simulink model "test_interp_method"  (R2025a)
settings: Solver=FixedStepAuto  StartTime=0.0  StopTime=.01  FixedStep=0.005  RelTol=1e-3
values from neighbouring files (symbols this model uses):
  SimIn =     [Model+Units_TEST.mat]    (also in SimIn_FROZEN.mat)
  ubar_cmd = 0.5 * (XU0_interp(1,4,2) + XU0_interp(1,3,2))    [config_and_run_interp_method_test.m]
  wbar_cmd = XU0_interp(3,3,2)    [config_and_run_interp_method_test.m]
libraries: simulink_extras x23
settings Model: Creator=alhallmark  LastModifiedBy=alhallmark

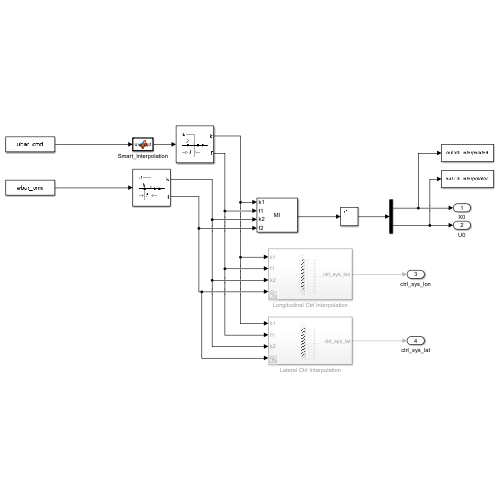
[thumbnail: Simulink's stored preview of the top-level diagram]
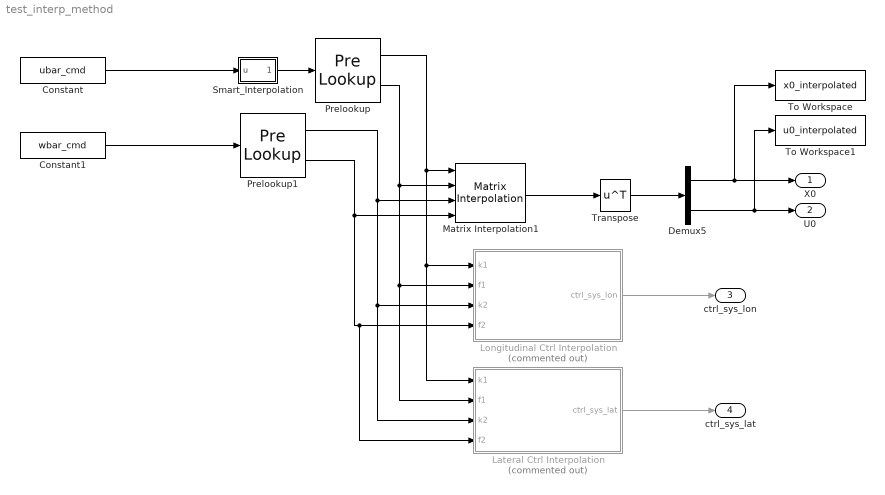
== system test_interp_method ==
  Constant : Constant  Value=ubar_cmd
  Constant1 : Constant  Value=wbar_cmd
  Demux5 : Demux  Outputs=[12 13]
  Lateral Ctrl Interpolation : Subsystem  Commented=on
  Longitudinal Ctrl Interpolation : Subsystem  Commented=on
  Matrix Interpolation1 : simulink_extras/Additional Lookup Tables/Matrix Interpolation  InterpMethod=Linear  ExtrapMethod=Clip  InterpolateDimension=2  TableData=SimIn.Control.trim.XU0_interp  SimulateUsing=Code generation
  Prelookup : PreLookup  BreakpointsData=SimIn.Control.trim.UH
  Prelookup1 : PreLookup  BreakpointsData=SimIn.Control.trim.WH
  Smart_Interpolation : MATLAB Function  TreatAsAtomicUnit=on
  To Workspace : ToWorkspace  VariableName=x0_interpolated  SampleTime=-1
  To Workspace1 : ToWorkspace  VariableName=u0_interpolated  SampleTime=-1
  Transpose : Math  Operator=transpose
  X0 : Outport
  U0 : Outport  Port=2
  ctrl_sys_lon : Outport  Port=3
  ctrl_sys_lat : Outport  Port=4
  wires:
  Longitudinal Ctrl Interpolation/1(ctrl_sys_lon) -> ctrl_sys_lon/1
  Constant/1 -> Smart_Interpolation/1(u)
  Demux5/1 -> To Workspace/1, X0/1
  Prelookup1/1 -> Longitudinal Ctrl Interpolation/3(k2), Lateral Ctrl Interpolation/3(k2), Matrix Interpolation1/3
  Prelookup/2 -> Longitudinal Ctrl Interpolation/2(f1), Lateral Ctrl Interpolation/2(f1), Matrix Interpolation1/2
  Demux5/2 -> U0/1, To Workspace1/1
  Transpose/1 -> Demux5/1
  Smart_Interpolation/1(u_out) -> Prelookup/1
  Prelookup1/2 -> Longitudinal Ctrl Interpolation/4(f2), Lateral Ctrl Interpolation/4(f2), Matrix Interpolation1/4
  Constant1/1 -> Prelookup1/1
  Prelookup/1 -> Matrix Interpolation1/1, Longitudinal Ctrl Interpolation/1(k1), Lateral Ctrl Interpolation/1(k1)
  Lateral Ctrl Interpolation/1(ctrl_sys_lat) -> ctrl_sys_lat/1
  Matrix Interpolation1/1 -> Transpose/1

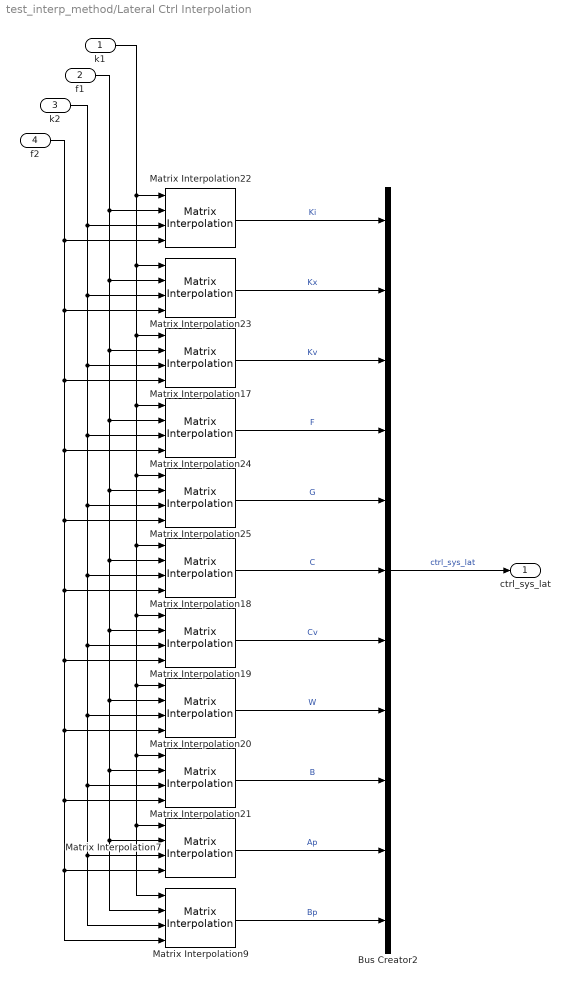
== system test_interp_method/Lateral Ctrl Interpolation ==
  k1 : Inport
  f1 : Inport  Port=2
  k2 : Inport  Port=3
  f2 : Inport  Port=4
  Bus Creator2 : BusCreator  Inputs=11
  Matrix Interpolation17 : simulink_extras/Additional Lookup Tables/Matrix Interpolation  InterpMethod=Linear  ExtrapMethod=Clip  InterpolateDimension=2  TableData=SimIn.Control.trim.Kv_lat_interp  SimulateUsing=Code generation
  Matrix Interpolation18 : simulink_extras/Additional Lookup Tables/Matrix Interpolation  InterpMethod=Linear  ExtrapMethod=Clip  InterpolateDimension=2  TableData=SimIn.Control.trim.C_lat_interp  SimulateUsing=Code generation
  Matrix Interpolation19 : simulink_extras/Additional Lookup Tables/Matrix Interpolation  InterpMethod=Linear  ExtrapMethod=Clip  InterpolateDimension=2  TableData=SimIn.Control.trim.Cv_lat_interp  SimulateUsing=Code generation
  Matrix Interpolation20 : simulink_extras/Additional Lookup Tables/Matrix Interpolation  InterpMethod=Linear  ExtrapMethod=Clip  InterpolateDimension=2  TableData=SimIn.Control.trim.W_lat_interp  SimulateUsing=Code generation
  Matrix Interpolation21 : simulink_extras/Additional Lookup Tables/Matrix Interpolation  InterpMethod=Linear  ExtrapMethod=Clip  InterpolateDimension=2  TableData=SimIn.Control.trim.B_lat_interp  SimulateUsing=Code generation
  Matrix Interpolation22 : simulink_extras/Additional Lookup Tables/Matrix Interpolation  InterpMethod=Linear  ExtrapMethod=Clip  InterpolateDimension=2  TableData=SimIn.Control.trim.Ki_lat_interp  SimulateUsing=Code generation
  Matrix Interpolation23 : simulink_extras/Additional Lookup Tables/Matrix Interpolation  InterpMethod=Linear  ExtrapMethod=Clip  InterpolateDimension=2  TableData=SimIn.Control.trim.Kx_lat_interp  SimulateUsing=Code generation
  Matrix Interpolation24 : simulink_extras/Additional Lookup Tables/Matrix Interpolation  InterpMethod=Linear  ExtrapMethod=Clip  InterpolateDimension=2  TableData=SimIn.Control.trim.F_lat_interp  SimulateUsing=Code generation
  Matrix Interpolation25 : simulink_extras/Additional Lookup Tables/Matrix Interpolation  InterpMethod=Linear  ExtrapMethod=Clip  InterpolateDimension=2  TableData=SimIn.Control.trim.G_lat_interp  SimulateUsing=Code generation
  Matrix Interpolation7 : simulink_extras/Additional Lookup Tables/Matrix Interpolation  InterpMethod=Linear  ExtrapMethod=Clip  InterpolateDimension=2  TableData=SimIn.Control.trim.Ap_lat_interp  SimulateUsing=Code generation
  Matrix Interpolation9 : simulink_extras/Additional Lookup Tables/Matrix Interpolation  InterpMethod=Linear  ExtrapMethod=Clip  InterpolateDimension=2  TableData=SimIn.Control.trim.Bp_lat_interp  SimulateUsing=Code generation
  ctrl_sys_lat : Outport
  wires:
  k1/1 -> Matrix Interpolation22/1, Matrix Interpolation23/1, Matrix Interpolation17/1, Matrix Interpolation25/1, Matrix Interpolation18/1, Matrix Interpolation19/1, Matrix Interpolation21/1, Matrix Interpolation9/1, Matrix Interpolation7/1, Matrix Interpolation20/1, Matrix Interpolation24/1
  k2/1 -> Matrix Interpolation22/3, Matrix Interpolation23/3, Matrix Interpolation17/3, Matrix Interpolation24/3, Matrix Interpolation25/3, Matrix Interpolation18/3, Matrix Interpolation19/3, Matrix Interpolation20/3, Matrix Interpolation21/3, Matrix Interpolation7/3, Matrix Interpolation9/3
  Matrix Interpolation20/1 -> Bus Creator2/8  "W"
  f2/1 -> Matrix Interpolation22/4, Matrix Interpolation23/4, Matrix Interpolation17/4, Matrix Interpolation24/4, Matrix Interpolation25/4, Matrix Interpolation18/4, Matrix Interpolation19/4, Matrix Interpolation20/4, Matrix Interpolation21/4, Matrix Interpolation7/4, Matrix Interpolation9/4
  f1/1 -> Matrix Interpolation22/2, Matrix Interpolation23/2, Matrix Interpolation17/2, Matrix Interpolation24/2, Matrix Interpolation25/2, Matrix Interpolation18/2, Matrix Interpolation19/2, Matrix Interpolation20/2, Matrix Interpolation21/2, Matrix Interpolation7/2, Matrix Interpolation9/2
  Matrix Interpolation22/1 -> Bus Creator2/1  "Ki"
  Matrix Interpolation17/1 -> Bus Creator2/3  "Kv"
  Matrix Interpolation18/1 -> Bus Creator2/6  "C"
  Matrix Interpolation19/1 -> Bus Creator2/7  "Cv"
  Matrix Interpolation23/1 -> Bus Creator2/2  "Kx"
  Matrix Interpolation9/1 -> Bus Creator2/11  "Bp"
  Matrix Interpolation25/1 -> Bus Creator2/5  "G"
  Matrix Interpolation24/1 -> Bus Creator2/4  "F"
  Matrix Interpolation21/1 -> Bus Creator2/9  "B"
  Matrix Interpolation7/1 -> Bus Creator2/10  "Ap"
  Bus Creator2/1 -> ctrl_sys_lat/1  "ctrl_sys_lat"

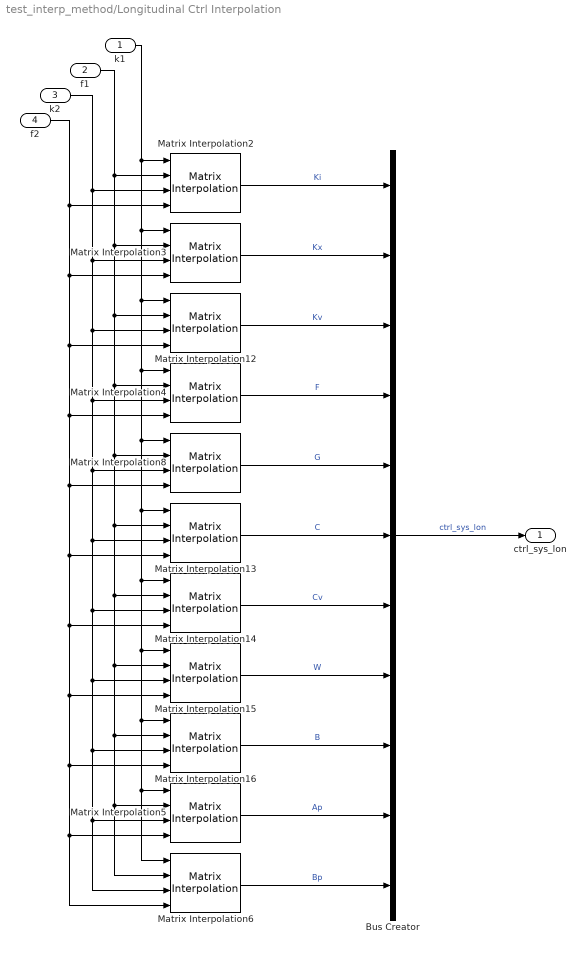
== system test_interp_method/Longitudinal Ctrl Interpolation ==
  k1 : Inport
  f1 : Inport  Port=2
  k2 : Inport  Port=3
  f2 : Inport  Port=4
  Bus Creator : BusCreator  Inputs=11
  Matrix Interpolation12 : simulink_extras/Additional Lookup Tables/Matrix Interpolation  InterpMethod=Linear  ExtrapMethod=Clip  InterpolateDimension=2  TableData=SimIn.Control.trim.Kv_lon_interp  SimulateUsing=Code generation
  Matrix Interpolation13 : simulink_extras/Additional Lookup Tables/Matrix Interpolation  InterpMethod=Linear  ExtrapMethod=Clip  InterpolateDimension=2  TableData=SimIn.Control.trim.C_lon_interp  SimulateUsing=Code generation
  Matrix Interpolation14 : simulink_extras/Additional Lookup Tables/Matrix Interpolation  InterpMethod=Linear  ExtrapMethod=Clip  InterpolateDimension=2  TableData=SimIn.Control.trim.Cv_lon_interp  SimulateUsing=Code generation
  Matrix Interpolation15 : simulink_extras/Additional Lookup Tables/Matrix Interpolation  InterpMethod=Linear  ExtrapMethod=Clip  InterpolateDimension=2  TableData=SimIn.Control.trim.W_lon_interp  SimulateUsing=Code generation
  Matrix Interpolation16 : simulink_extras/Additional Lookup Tables/Matrix Interpolation  InterpMethod=Linear  ExtrapMethod=Clip  InterpolateDimension=2  TableData=SimIn.Control.trim.B_lon_interp  SimulateUsing=Code generation
  Matrix Interpolation2 : simulink_extras/Additional Lookup Tables/Matrix Interpolation  InterpMethod=Linear  ExtrapMethod=Clip  InterpolateDimension=2  TableData=SimIn.Control.trim.Ki_lon_interp  SimulateUsing=Code generation
  Matrix Interpolation3 : simulink_extras/Additional Lookup Tables/Matrix Interpolation  InterpMethod=Linear  ExtrapMethod=Clip  InterpolateDimension=2  TableData=SimIn.Control.trim.Kx_lon_interp  SimulateUsing=Code generation
  Matrix Interpolation4 : simulink_extras/Additional Lookup Tables/Matrix Interpolation  InterpMethod=Linear  ExtrapMethod=Clip  InterpolateDimension=2  TableData=SimIn.Control.trim.F_lon_interp  SimulateUsing=Code generation
  Matrix Interpolation5 : simulink_extras/Additional Lookup Tables/Matrix Interpolation  InterpMethod=Linear  ExtrapMethod=Clip  InterpolateDimension=2  TableData=SimIn.Control.trim.Ap_lon_interp  SimulateUsing=Code generation
  Matrix Interpolation6 : simulink_extras/Additional Lookup Tables/Matrix Interpolation  InterpMethod=Linear  ExtrapMethod=Clip  InterpolateDimension=2  TableData=SimIn.Control.trim.Bp_lon_interp  SimulateUsing=Code generation
  Matrix Interpolation8 : simulink_extras/Additional Lookup Tables/Matrix Interpolation  InterpMethod=Linear  ExtrapMethod=Clip  InterpolateDimension=2  TableData=SimIn.Control.trim.G_lon_interp  SimulateUsing=Code generation
  ctrl_sys_lon : Outport
  wires:
  f1/1 -> Matrix Interpolation2/2, Matrix Interpolation3/2, Matrix Interpolation12/2, Matrix Interpolation4/2, Matrix Interpolation8/2, Matrix Interpolation13/2, Matrix Interpolation14/2, Matrix Interpolation15/2, Matrix Interpolation16/2, Matrix Interpolation5/2, Matrix Interpolation6/2
  Matrix Interpolation6/1 -> Bus Creator/11  "Bp"
  k2/1 -> Matrix Interpolation2/3, Matrix Interpolation3/3, Matrix Interpolation12/3, Matrix Interpolation4/3, Matrix Interpolation8/3, Matrix Interpolation13/3, Matrix Interpolation14/3, Matrix Interpolation15/3, Matrix Interpolation16/3, Matrix Interpolation5/3, Matrix Interpolation6/3
  k1/1 -> Matrix Interpolation2/1, Matrix Interpolation3/1, Matrix Interpolation12/1, Matrix Interpolation4/1, Matrix Interpolation8/1, Matrix Interpolation13/1, Matrix Interpolation14/1, Matrix Interpolation15/1, Matrix Interpolation5/1, Matrix Interpolation6/1, Matrix Interpolation16/1
  Matrix Interpolation3/1 -> Bus Creator/2  "Kx"
  Matrix Interpolation13/1 -> Bus Creator/6  "C"
  Matrix Interpolation8/1 -> Bus Creator/5  "G"
  Matrix Interpolation16/1 -> Bus Creator/9  "B"
  Matrix Interpolation2/1 -> Bus Creator/1  "Ki"
  Matrix Interpolation14/1 -> Bus Creator/7  "Cv"
  Matrix Interpolation4/1 -> Bus Creator/4  "F"
  Matrix Interpolation5/1 -> Bus Creator/10  "Ap"
  Matrix Interpolation15/1 -> Bus Creator/8  "W"
  Matrix Interpolation12/1 -> Bus Creator/3  "Kv"
  Bus Creator/1 -> ctrl_sys_lon/1  "ctrl_sys_lon"
  f2/1 -> Matrix Interpolation2/4, Matrix Interpolation3/4, Matrix Interpolation12/4, Matrix Interpolation4/4, Matrix Interpolation8/4, Matrix Interpolation13/4, Matrix Interpolation14/4, Matrix Interpolation15/4, Matrix Interpolation16/4, Matrix Interpolation5/4, Matrix Interpolation6/4

== matlab function test_interp_method/Smart_Interpolation ==
  data: u input; u_out output
function u_out = fcn(u)

% This function is used to limit interpolation for three portions of the
% flight envelope: 1) Below zero knots, 2) After the end of transition
% (90 kts) and before cruise (100 knots) and 3) above the last trim map
% point (130 knots)

ft2kts = 0.3048/1852.0*3600; % Conversion factor of ft/sec to knots (derived from setUnits values)
kts2ft = 1/ft2kts; % Conversion factor from knots to ft/sec
if u < 0* kts2ft; % SimIn.Control.trim.UH(1)
    u_out = 0*kts2ft; % SimIn.Control.trim.UH(1);
% elseif u>90*kts2ft && u<100*kts2ft
%     u_out = 100*kts2ft;
elseif u>130*kts2ft % SimIn.Control.trim.UH(end)
    u_out = 130*kts2ft; % SimIn.Control.trim.UH(end)
else
    u_out = u;
end
